simulink model "propeller"  (R2019b)
settings: Solver=VariableStepAuto  StartTime=0.0  StopTime=180  MaxStep=1e-2  RelTol=1e-3
undefined symbols (not defined in the file or in its folder): X, Y, Z
libraries: sm_lib x26, cstblocks x23, nesl_utility x20, simulink x2
(part 2 of 3)

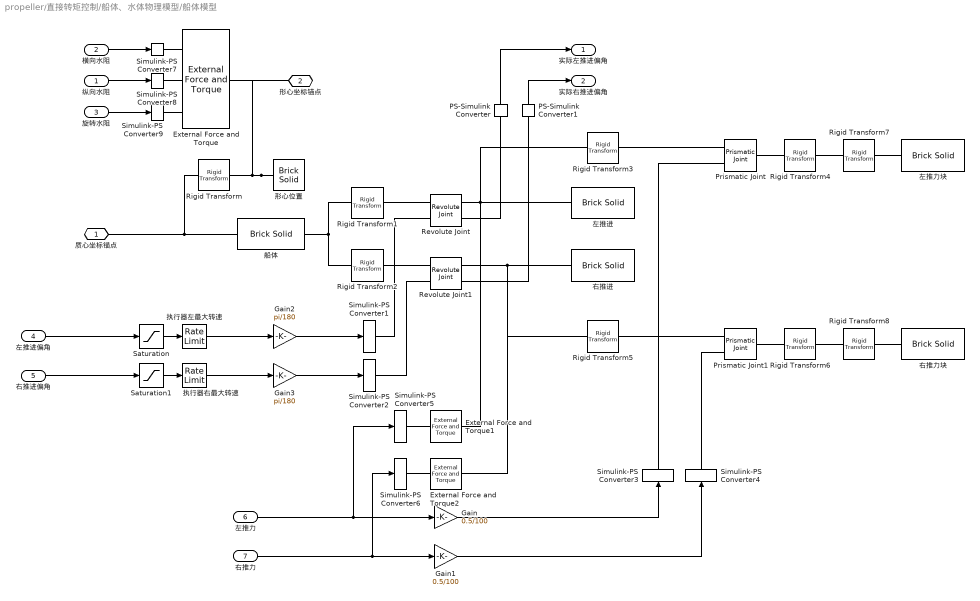
== system propeller/直接转矩控制/船体、水体物理模型/船体模型 ==
  纵向水阻 : Inport
  横向水阻 : Inport  Port=2
  旋转水阻 : Inport  Port=3
  左推进偏角 : Inport  Port=4
  右推进偏角 : Inport  Port=5
  左推力 : Inport  Port=6
  右推力 : Inport  Port=7
  External Force and Torque : sm_lib/Forces and Torques/External Force and Torque  ForceResolutionFrame=AttachedFrame  EnableForceX=on  EnableForceY=on  EnableForceZ=off  EnableForce=off  TorqueResolutionFrame=AttachedFrame  EnableTorqueX=off  EnableTorqueY=off  EnableTorqueZ=on  EnableTorque=off
  External Force and Torque1 : sm_lib/Forces and Torques/External Force and Torque  ForceResolutionFrame=AttachedFrame  EnableForceX=off  EnableForceY=on  EnableForceZ=off  EnableForce=off  TorqueResolutionFrame=AttachedFrame  EnableTorqueX=off  EnableTorqueY=off  EnableTorqueZ=off  EnableTorque=off
  External Force and Torque2 : sm_lib/Forces and Torques/External Force and Torque  ForceResolutionFrame=AttachedFrame  EnableForceX=off  EnableForceY=on  EnableForceZ=off  EnableForce=off  TorqueResolutionFrame=AttachedFrame  EnableTorqueX=off  EnableTorqueY=off  EnableTorqueZ=off  EnableTorque=off
  Gain : Gain  Gain=0.5/100
  Gain1 : Gain  Gain=0.5/100
  Gain2 : Gain  Gain=pi/180
  Gain3 : Gain  Gain=pi/180
  PS-Simulink Converter : nesl_utility/PS-Simulink Converter  PhysicalDomain=network_engine_domain  SubClassName=ps_output  LeftPortType=input  RightPortType=output  PseudoPeriodic=off  Frequencies=[]  Unit=inherit  AffineConversion=off
  PS-Simulink Converter1 : nesl_utility/PS-Simulink Converter  PhysicalDomain=network_engine_domain  SubClassName=ps_output  LeftPortType=input  RightPortType=output  PseudoPeriodic=off  Frequencies=[]  Unit=inherit  AffineConversion=off
  Prismatic Joint : sm_lib/Joints/Prismatic Joint  JointMode=Normal  SenseConstraintForce=off  SenseConstraintForceX=off  SenseConstraintForceY=off  SenseConstraintForceZ=off  SenseConstraintTorque=off  SenseConstraintTorqueX=off  SenseConstraintTorqueY=off  SenseConstraintTorqueZ=off  SenseTotalForce=off  SenseTotalForceX=off  SenseTotalForceY=off  SenseTotalForceZ=off  SenseTotalTorque=off  SenseTotalTorqueX=off  SenseTotalTorqueY=off  SenseTotalTorqueZ=off  CompositeWrenchDir=FollowerOnBase  CompositeWrenchFrame=BaseFrame  EquilibriumPosition=0  EquilibriumPositionUnits=m  SpringStiffness=0  SpringStiffnessUnits=N/m  DampingCoefficient=0  DampingCoefficientUnits=N/(m/s)  TorqueActuationMode=ComputedTorque  MotionActuationMode=InputMotion  SensePosition=off  SenseVelocity=off  SenseAcceleration=off  SenseTorqueForce=off  SenseLowerLimitTorqueForce=off  SenseUpperLimitTorqueForce=off  LowerLimitSpecify=off  LowerLimitBound=-1  LowerLimitBoundUnits=m  LowerLimitStiffness=1e6  LowerLimitStiffnessUnits=N/m  LowerLimitDamping=1e3  LowerLimitDampingUnits=N/(m/s)  LowerLimitTransitionRegionWidth=1e-4  LowerLimitTransitionRegionWidthUnits=m  UpperLimitSpecify=off  UpperLimitBound=1  UpperLimitBoundUnits=m  UpperLimitStiffness=1e6  UpperLimitStiffnessUnits=N/m  UpperLimitDamping=1e3  UpperLimitDampingUnits=N/(m/s)  UpperLimitTransitionRegionWidth=1e-4  UpperLimitTransitionRegionWidthUnits=m  PositionTargetSpecify=off  PositionTargetPriority=High  PositionTargetValue=0  PositionTargetValueUnits=m  VelocityTargetSpecify=off  VelocityTargetPriority=High  VelocityTargetValue=0  VelocityTargetValueUnits=m/s
  Prismatic Joint1 : sm_lib/Joints/Prismatic Joint  JointMode=Normal  SenseConstraintForce=off  SenseConstraintForceX=off  SenseConstraintForceY=off  SenseConstraintForceZ=off  SenseConstraintTorque=off  SenseConstraintTorqueX=off  SenseConstraintTorqueY=off  SenseConstraintTorqueZ=off  SenseTotalForce=off  SenseTotalForceX=off  SenseTotalForceY=off  SenseTotalForceZ=off  SenseTotalTorque=off  SenseTotalTorqueX=off  SenseTotalTorqueY=off  SenseTotalTorqueZ=off  CompositeWrenchDir=FollowerOnBase  CompositeWrenchFrame=BaseFrame  EquilibriumPosition=0  EquilibriumPositionUnits=m  SpringStiffness=0  SpringStiffnessUnits=N/m  DampingCoefficient=0  DampingCoefficientUnits=N/(m/s)  TorqueActuationMode=ComputedTorque  MotionActuationMode=InputMotion  SensePosition=off  SenseVelocity=off  SenseAcceleration=off  SenseTorqueForce=off  SenseLowerLimitTorqueForce=off  SenseUpperLimitTorqueForce=off  LowerLimitSpecify=off  LowerLimitBound=-1  LowerLimitBoundUnits=m  LowerLimitStiffness=1e6  LowerLimitStiffnessUnits=N/m  LowerLimitDamping=1e3  LowerLimitDampingUnits=N/(m/s)  LowerLimitTransitionRegionWidth=1e-4  LowerLimitTransitionRegionWidthUnits=m  UpperLimitSpecify=off  UpperLimitBound=1  UpperLimitBoundUnits=m  UpperLimitStiffness=1e6  UpperLimitStiffnessUnits=N/m  UpperLimitDamping=1e3  UpperLimitDampingUnits=N/(m/s)  UpperLimitTransitionRegionWidth=1e-4  UpperLimitTransitionRegionWidthUnits=m  PositionTargetSpecify=off  PositionTargetPriority=High  PositionTargetValue=0  PositionTargetValueUnits=m  VelocityTargetSpecify=off  VelocityTargetPriority=High  VelocityTargetValue=0  VelocityTargetValueUnits=m/s
  Revolute Joint : sm_lib/Joints/Revolute Joint  JointMode=Normal  SenseConstraintForce=off  SenseConstraintForceX=off  SenseConstraintForceY=off  SenseConstraintForceZ=off  SenseConstraintTorque=off  SenseConstraintTorqueX=off  SenseConstraintTorqueY=off  SenseConstraintTorqueZ=off  SenseTotalForce=off  SenseTotalForceX=off  SenseTotalForceY=off  SenseTotalForceZ=off  SenseTotalTorque=off  SenseTotalTorqueX=off  SenseTotalTorqueY=off  SenseTotalTorqueZ=off  CompositeWrenchDir=FollowerOnBase  CompositeWrenchFrame=BaseFrame  EquilibriumPosition=0  EquilibriumPositionUnits=deg  SpringStiffness=0  SpringStiffnessUnits=N*m/deg  DampingCoefficient=0  DampingCoefficientUnits=N*m/(deg/s)  TorqueActuationMode=ComputedTorque  MotionActuationMode=InputMotion  SensePosition=on  SenseVelocity=off  SenseAcceleration=off  SenseTorqueForce=off  SenseLowerLimitTorqueForce=off  SenseUpperLimitTorqueForce=off  LowerLimitSpecify=off  LowerLimitBound=-90  LowerLimitBoundUnits=deg  LowerLimitStiffness=1e4  LowerLimitStiffnessUnits=N*m/deg  LowerLimitDamping=10  LowerLimitDampingUnits=N*m/(deg/s)  LowerLimitTransitionRegionWidth=0.1  LowerLimitTransitionRegionWidthUnits=deg  UpperLimitSpecify=off  UpperLimitBound=90  UpperLimitBoundUnits=deg  UpperLimitStiffness=1e4  UpperLimitStiffnessUnits=N*m/deg  UpperLimitDamping=10  UpperLimitDampingUnits=N*m/(deg/s)  UpperLimitTransitionRegionWidth=0.1  UpperLimitTransitionRegionWidthUnits=deg  PositionTargetSpecify=off  PositionTargetPriority=High  PositionTargetValue=0  PositionTargetValueUnits=deg  VelocityTargetSpecify=off  VelocityTargetPriority=High  VelocityTargetValue=0  VelocityTargetValueUnits=deg/s
  Revolute Joint1 : sm_lib/Joints/Revolute Joint  JointMode=Normal  SenseConstraintForce=off  SenseConstraintForceX=off  SenseConstraintForceY=off  SenseConstraintForceZ=off  SenseConstraintTorque=off  SenseConstraintTorqueX=off  SenseConstraintTorqueY=off  SenseConstraintTorqueZ=off  SenseTotalForce=off  SenseTotalForceX=off  SenseTotalForceY=off  SenseTotalForceZ=off  SenseTotalTorque=off  SenseTotalTorqueX=off  SenseTotalTorqueY=off  SenseTotalTorqueZ=off  CompositeWrenchDir=FollowerOnBase  CompositeWrenchFrame=BaseFrame  EquilibriumPosition=0  EquilibriumPositionUnits=deg  SpringStiffness=0  SpringStiffnessUnits=N*m/deg  DampingCoefficient=0  DampingCoefficientUnits=N*m/(deg/s)  TorqueActuationMode=ComputedTorque  MotionActuationMode=InputMotion  SensePosition=on  SenseVelocity=off  SenseAcceleration=off  SenseTorqueForce=off  SenseLowerLimitTorqueForce=off  SenseUpperLimitTorqueForce=off  LowerLimitSpecify=off  LowerLimitBound=-90  LowerLimitBoundUnits=deg  LowerLimitStiffness=1e4  LowerLimitStiffnessUnits=N*m/deg  LowerLimitDamping=10  LowerLimitDampingUnits=N*m/(deg/s)  LowerLimitTransitionRegionWidth=0.1  LowerLimitTransitionRegionWidthUnits=deg  UpperLimitSpecify=off  UpperLimitBound=90  UpperLimitBoundUnits=deg  UpperLimitStiffness=1e4  UpperLimitStiffnessUnits=N*m/deg  UpperLimitDamping=10  UpperLimitDampingUnits=N*m/(deg/s)  UpperLimitTransitionRegionWidth=0.1  UpperLimitTransitionRegionWidthUnits=deg  PositionTargetSpecify=off  PositionTargetPriority=High  PositionTargetValue=0  PositionTargetValueUnits=deg  VelocityTargetSpecify=off  VelocityTargetPriority=High  VelocityTargetValue=0  VelocityTargetValueUnits=deg/s
  Rigid Transform : sm_lib/Frames and Transforms/Rigid Transform  TranslationMethod=Cartesian  TranslationStandardOffset=1  TranslationLengthUnit=m  TranslationStandardAxis=-Y  TranslationCartesianOffset=[0 -1 0]  TranslationROffset=0  TranslationROffsetUnits=m  TranslationZOffset=0  TranslationZOffsetUnits=m  TranslationThetaOffset=0  TranslationThetaOffsetUnits=deg  RotationMethod=None  RotationAngleUnits=deg  RotationStandardAxis=+Z  RotationAngle=0.0  RotationArbitraryAxis=[0 0 1]  FollAlignAxisA=+X  BaseAlignAxisA=+Y  FollAlignAxisB=+Y  BaseAlignAxisB=+Z  RotationSequenceAxes=FollowerAxes  RotationSequence=XYX  RotationSequenceAngles=[0 0 0]  RotationSequenceAnglesUnits=deg  RotationMatrix=[1 0 0; 0 1 0; 0 0 1]
  Rigid Transform1 : sm_lib/Frames and Transforms/Rigid Transform  TranslationMethod=Cartesian  TranslationStandardOffset=1  TranslationLengthUnit=m  TranslationStandardAxis=-Y  TranslationCartesianOffset=[-1 0 0]  TranslationROffset=0  TranslationROffsetUnits=m  TranslationZOffset=0  TranslationZOffsetUnits=m  TranslationThetaOffset=0  TranslationThetaOffsetUnits=deg  RotationMethod=None  RotationAngleUnits=deg  RotationStandardAxis=+Z  RotationAngle=0.0  RotationArbitraryAxis=[0 0 1]  FollAlignAxisA=+X  BaseAlignAxisA=+Y  FollAlignAxisB=+Y  BaseAlignAxisB=+Z  RotationSequenceAxes=FollowerAxes  RotationSequence=XYX  RotationSequenceAngles=[0 0 0]  RotationSequenceAnglesUnits=deg  RotationMatrix=[1 0 0; 0 1 0; 0 0 1]
  Rigid Transform2 : sm_lib/Frames and Transforms/Rigid Transform  TranslationMethod=Cartesian  TranslationStandardOffset=1  TranslationLengthUnit=m  TranslationStandardAxis=-Y  TranslationCartesianOffset=[1 0 0]  TranslationROffset=0  TranslationROffsetUnits=m  TranslationZOffset=0  TranslationZOffsetUnits=m  TranslationThetaOffset=0  TranslationThetaOffsetUnits=deg  RotationMethod=None  RotationAngleUnits=deg  RotationStandardAxis=+Z  RotationAngle=0.0  RotationArbitraryAxis=[0 0 1]  FollAlignAxisA=+X  BaseAlignAxisA=+Y  FollAlignAxisB=+Y  BaseAlignAxisB=+Z  RotationSequenceAxes=FollowerAxes  RotationSequence=XYX  RotationSequenceAngles=[0 0 0]  RotationSequenceAnglesUnits=deg  RotationMatrix=[1 0 0; 0 1 0; 0 0 1]
  Rigid Transform3 : sm_lib/Frames and Transforms/Rigid Transform  TranslationMethod=None  TranslationStandardOffset=1  TranslationLengthUnit=m  TranslationStandardAxis=-Y  TranslationCartesianOffset=[0 -1 0]  TranslationROffset=0  TranslationROffsetUnits=m  TranslationZOffset=0  TranslationZOffsetUnits=m  TranslationThetaOffset=0  TranslationThetaOffsetUnits=deg  RotationMethod=StandardAxis  RotationAngleUnits=deg  RotationStandardAxis=+X  RotationAngle=90  RotationArbitraryAxis=[0 0 1]  FollAlignAxisA=+X  BaseAlignAxisA=+Y  FollAlignAxisB=+Y  BaseAlignAxisB=+Z  RotationSequenceAxes=FollowerAxes  RotationSequence=XYX  RotationSequenceAngles=[0 0 0]  RotationSequenceAnglesUnits=deg  RotationMatrix=[1 0 0; 0 1 0; 0 0 1]
  Rigid Transform4 : sm_lib/Frames and Transforms/Rigid Transform  TranslationMethod=None  TranslationStandardOffset=1  TranslationLengthUnit=m  TranslationStandardAxis=-Y  TranslationCartesianOffset=[0 -1 0]  TranslationROffset=0  TranslationROffsetUnits=m  TranslationZOffset=0  TranslationZOffsetUnits=m  TranslationThetaOffset=0  TranslationThetaOffsetUnits=deg  RotationMethod=StandardAxis  RotationAngleUnits=deg  RotationStandardAxis=-X  RotationAngle=90  RotationArbitraryAxis=[0 0 1]  FollAlignAxisA=+X  BaseAlignAxisA=+Y  FollAlignAxisB=+Y  BaseAlignAxisB=+Z  RotationSequenceAxes=FollowerAxes  RotationSequence=XYX  RotationSequenceAngles=[0 0 0]  RotationSequenceAnglesUnits=deg  RotationMatrix=[1 0 0; 0 1 0; 0 0 1]
  Rigid Transform5 : sm_lib/Frames and Transforms/Rigid Transform  TranslationMethod=None  TranslationStandardOffset=1  TranslationLengthUnit=m  TranslationStandardAxis=-Y  TranslationCartesianOffset=[0 -1 0]  TranslationROffset=0  TranslationROffsetUnits=m  TranslationZOffset=0  TranslationZOffsetUnits=m  TranslationThetaOffset=0  TranslationThetaOffsetUnits=deg  RotationMethod=StandardAxis  RotationAngleUnits=deg  RotationStandardAxis=+X  RotationAngle=90  RotationArbitraryAxis=[0 0 1]  FollAlignAxisA=+X  BaseAlignAxisA=+Y  FollAlignAxisB=+Y  BaseAlignAxisB=+Z  RotationSequenceAxes=FollowerAxes  RotationSequence=XYX  RotationSequenceAngles=[0 0 0]  RotationSequenceAnglesUnits=deg  RotationMatrix=[1 0 0; 0 1 0; 0 0 1]
  Rigid Transform6 : sm_lib/Frames and Transforms/Rigid Transform  TranslationMethod=None  TranslationStandardOffset=1  TranslationLengthUnit=m  TranslationStandardAxis=-Y  TranslationCartesianOffset=[0 -1 0]  TranslationROffset=0  TranslationROffsetUnits=m  TranslationZOffset=0  TranslationZOffsetUnits=m  TranslationThetaOffset=0  TranslationThetaOffsetUnits=deg  RotationMethod=StandardAxis  RotationAngleUnits=deg  RotationStandardAxis=-X  RotationAngle=90  RotationArbitraryAxis=[0 0 1]  FollAlignAxisA=+X  BaseAlignAxisA=+Y  FollAlignAxisB=+Y  BaseAlignAxisB=+Z  RotationSequenceAxes=FollowerAxes  RotationSequence=XYX  RotationSequenceAngles=[0 0 0]  RotationSequenceAnglesUnits=deg  RotationMatrix=[1 0 0; 0 1 0; 0 0 1]
  Rigid Transform7 : sm_lib/Frames and Transforms/Rigid Transform  TranslationMethod=StandardAxis  TranslationStandardOffset=0.25  TranslationLengthUnit=m  TranslationStandardAxis=-Y  TranslationCartesianOffset=[0 -1 0]  TranslationROffset=0  TranslationROffsetUnits=m  TranslationZOffset=0  TranslationZOffsetUnits=m  TranslationThetaOffset=0  TranslationThetaOffsetUnits=deg  RotationMethod=None  RotationAngleUnits=deg  RotationStandardAxis=-X  RotationAngle=90  RotationArbitraryAxis=[0 0 1]  FollAlignAxisA=+X  BaseAlignAxisA=+Y  FollAlignAxisB=+Y  BaseAlignAxisB=+Z  RotationSequenceAxes=FollowerAxes  RotationSequence=XYX  RotationSequenceAngles=[0 0 0]  RotationSequenceAnglesUnits=deg  RotationMatrix=[1 0 0; 0 1 0; 0 0 1]
  Rigid Transform8 : sm_lib/Frames and Transforms/Rigid Transform  TranslationMethod=StandardAxis  TranslationStandardOffset=0.25  TranslationLengthUnit=m  TranslationStandardAxis=-Y  TranslationCartesianOffset=[0 -1 0]  TranslationROffset=0  TranslationROffsetUnits=m  TranslationZOffset=0  TranslationZOffsetUnits=m  TranslationThetaOffset=0  TranslationThetaOffsetUnits=deg  RotationMethod=None  RotationAngleUnits=deg  RotationStandardAxis=-X  RotationAngle=90  RotationArbitraryAxis=[0 0 1]  FollAlignAxisA=+X  BaseAlignAxisA=+Y  FollAlignAxisB=+Y  BaseAlignAxisB=+Z  RotationSequenceAxes=FollowerAxes  RotationSequence=XYX  RotationSequenceAngles=[0 0 0]  RotationSequenceAnglesUnits=deg  RotationMatrix=[1 0 0; 0 1 0; 0 0 1]
  Saturation : Saturate  UpperLimit=30  LowerLimit=-30
  Saturation1 : Saturate  UpperLimit=30  LowerLimit=-30
  Simulink-PS Converter{1..4} (4 alike) : nesl_utility/Simulink-PS Converter  PhysicalDomain=network_engine_domain  SubClassName=ps_input  LeftPortType=input  RightPortType=output  PseudoPeriodic=off  Frequencies=[]  NoiseDistribution=none  NoiseParameters=[]  Unit=1  AffineConversion=off  FilteringAndDerivatives=filter  SimscapeFilterOrder=2  InputFilterTimeConstant=0.01  UdotUserProvided=1
  Simulink-PS Converter{5..9} (5 alike) : nesl_utility/Simulink-PS Converter  PhysicalDomain=network_engine_domain  SubClassName=ps_input  LeftPortType=input  RightPortType=output  PseudoPeriodic=off  Frequencies=[]  NoiseDistribution=none  NoiseParameters=[]  Unit=1  AffineConversion=off  FilteringAndDerivatives=provide  SimscapeFilterOrder=2  InputFilterTimeConstant=0.01  UdotUserProvided=0
  右推力块 : sm_lib/Body Elements/Brick Solid  GraphicAmbientColor=[0.15 0.15 0.15 1.0]  BasedOnType=Mass  BrickDimensions=[0.15 0.05 0.15]  BrickDimensionUnits=m  CenterOfMass=[0 0 0]  CenterOfMassUnits=m  GraphicDiffuseColor=[0.8 0.0 0.0]  Density=1000  DensityUnits=kg/m^3  DoExposeReferenceFrame=off  GraphicEmissiveColor=[0.0 0.0 0.0 1.0]  ExportEntireGeometry=off  SerializedFrames=<Frames><Frame><Id>Frame1</Id><Value><Name>零位面</Name><Origin><Source>CenterOfMassFrame</Source><FeatureName></FeatureName></Origin><PrimaryAxis><DefinedDirection>+Z</DefinedDirection><Source>ReferenceFrame</Source><SourceDirection>+Z</SourceDirection><FeatureName></FeatureName></PrimaryAxis><SecondaryAxis><DefinedDirection>+X</DefinedDirection><Source>ReferenceFrame</Source><SourceDirection>+X</SourceDirection><FeatureName></FeatureName></SecondaryAxis></Value></Frame></Frames>  MarkerShape=Sphere  MarkerSize=10  GraphicType=FromGeometry  InertiaType=CalculateFromGeometry  Mass=0  MassUnits=kg  MomentsOfInertia=[1 1 1]  MomentsOfInertiaUnits=kg*m^2  GraphicOpacity=1  ProductsOfInertia=[0 0 0]  ProductsOfInertiaUnits=kg*m^2  GraphicShininess=75  GraphicSpecularColor=[0.5 0.5 0.5 1.0]  GraphicVisPropType=SimpleVisualProperties
  右推进 : sm_lib/Body Elements/Brick Solid  GraphicAmbientColor=[0.15 0.15 0.15 1.0]  BasedOnType=Mass  BrickDimensions=[0.2 0.5 0.2]  BrickDimensionUnits=m  CenterOfMass=[0 0 0]  CenterOfMassUnits=m  GraphicDiffuseColor=[0.6 0.6 1.0]  Density=1000  DensityUnits=kg/m^3  DoExposeReferenceFrame=off  GraphicEmissiveColor=[0.0 0.0 0.0 1.0]  ExportEntireGeometry=off  SerializedFrames=<Frames><Frame><Id>Frame1</Id><Value><Name>转轴</Name><Origin><Source>GeometricFeature</Source><FeatureName>+y surface</FeatureName></Origin><PrimaryAxis><DefinedDirection>+Z</DefinedDirection><Source>ReferenceFrame</Source><SourceDirection>+Z</SourceDirection><FeatureName></FeatureName></PrimaryAxis><SecondaryAxis><DefinedDirection>+X</DefinedDirection><Source>ReferenceFrame</Source><SourceDirection>+X</SourceDirection><FeatureName></FeatureName></SecondaryAxis></Value></Frame></Frames>  MarkerShape=Sphere  MarkerSize=10  GraphicType=FromGeometry  InertiaType=CalculateFromGeometry  Mass=0  MassUnits=kg  MomentsOfInertia=[1 1 1]  MomentsOfInertiaUnits=kg*m^2  GraphicOpacity=0.3  ProductsOfInertia=[0 0 0]  ProductsOfInertiaUnits=kg*m^2  GraphicShininess=75  GraphicSpecularColor=[0.5 0.5 0.5 1.0]  GraphicVisPropType=SimpleVisualProperties
  左推力块 : sm_lib/Body Elements/Brick Solid  GraphicAmbientColor=[0.15 0.15 0.15 1.0]  BasedOnType=Mass  BrickDimensions=[0.15 0.05 0.15]  BrickDimensionUnits=m  CenterOfMass=[0 0 0]  CenterOfMassUnits=m  GraphicDiffuseColor=[0.8 0.0 0.0]  Density=1000  DensityUnits=kg/m^3  DoExposeReferenceFrame=off  GraphicEmissiveColor=[0.0 0.0 0.0 1.0]  ExportEntireGeometry=off  SerializedFrames=<Frames><Frame><Id>Frame1</Id><Value><Name>零位面</Name><Origin><Source>CenterOfMassFrame</Source><FeatureName></FeatureName></Origin><PrimaryAxis><DefinedDirection>+Z</DefinedDirection><Source>ReferenceFrame</Source><SourceDirection>+Z</SourceDirection><FeatureName></FeatureName></PrimaryAxis><SecondaryAxis><DefinedDirection>+X</DefinedDirection><Source>ReferenceFrame</Source><SourceDirection>+X</SourceDirection><FeatureName></FeatureName></SecondaryAxis></Value></Frame></Frames>  MarkerShape=Sphere  MarkerSize=10  GraphicType=FromGeometry  InertiaType=CalculateFromGeometry  Mass=0  MassUnits=kg  MomentsOfInertia=[1 1 1]  MomentsOfInertiaUnits=kg*m^2  GraphicOpacity=1  ProductsOfInertia=[0 0 0]  ProductsOfInertiaUnits=kg*m^2  GraphicShininess=75  GraphicSpecularColor=[0.5 0.5 0.5 1.0]  GraphicVisPropType=SimpleVisualProperties
  左推进 : sm_lib/Body Elements/Brick Solid  GraphicAmbientColor=[0.15 0.15 0.15 1.0]  BasedOnType=Mass  BrickDimensions=[0.2 0.5 0.2]  BrickDimensionUnits=m  CenterOfMass=[0 0 0]  CenterOfMassUnits=m  GraphicDiffuseColor=[0.6 0.6 1.0]  Density=1000  DensityUnits=kg/m^3  DoExposeReferenceFrame=off  GraphicEmissiveColor=[0.0 0.0 0.0 1.0]  ExportEntireGeometry=off  SerializedFrames=<Frames><Frame><Id>Frame1</Id><Value><Name>转轴</Name><Origin><Source>GeometricFeature</Source><FeatureName>+y surface</FeatureName></Origin><PrimaryAxis><DefinedDirection>+Z</DefinedDirection><Source>ReferenceFrame</Source><SourceDirection>+Z</SourceDirection><FeatureName></FeatureName></PrimaryAxis><SecondaryAxis><DefinedDirection>+X</DefinedDirection><Source>ReferenceFrame</Source><SourceDirection>+X</SourceDirection><FeatureName></FeatureName></SecondaryAxis></Value></Frame></Frames>  MarkerShape=Sphere  MarkerSize=10  GraphicType=FromGeometry  InertiaType=CalculateFromGeometry  Mass=0  MassUnits=kg  MomentsOfInertia=[1 1 1]  MomentsOfInertiaUnits=kg*m^2  GraphicOpacity=0.3  ProductsOfInertia=[0 0 0]  ProductsOfInertiaUnits=kg*m^2  GraphicShininess=75  GraphicSpecularColor=[0.5 0.5 0.5 1.0]  GraphicVisPropType=SimpleVisualProperties
  形心位置 : sm_lib/Body Elements/Brick Solid  GraphicAmbientColor=[0.15 0.15 0.15 1.0]  BasedOnType=Mass  BrickDimensions=[0.2 0.2 0.2]  BrickDimensionUnits=m  CenterOfMass=[0 0 0]  CenterOfMassUnits=m  GraphicDiffuseColor=[0.0 0.0 0.8]  Density=1000  DensityUnits=kg/m^3  DoExposeReferenceFrame=on  GraphicEmissiveColor=[0.0 0.0 0.0 1.0]  ExportEntireGeometry=off  SerializedFrames=<Frames/>  MarkerShape=Sphere  MarkerSize=10  GraphicType=FromGeometry  InertiaType=CalculateFromGeometry  Mass=0  MassUnits=kg  MomentsOfInertia=[1 1 1]  MomentsOfInertiaUnits=kg*m^2  GraphicOpacity=0.8  ProductsOfInertia=[0 0 0]  ProductsOfInertiaUnits=kg*m^2  GraphicShininess=75  GraphicSpecularColor=[0.5 0.5 0.5 1.0]  GraphicVisPropType=SimpleVisualProperties
  执行器右最大转速 : RateLimiter  RisingSlewLimit=15  FallingSlewLimit=-15  SampleTimeMode=inherited
  执行器左最大转速 : RateLimiter  RisingSlewLimit=15  FallingSlewLimit=-15  SampleTimeMode=inherited
  船体 : sm_lib/Body Elements/Brick Solid  GraphicAmbientColor=[0.15 0.15 0.15 1.0]  BasedOnType=Mass  BrickDimensions=[3 6 0.5]  BrickDimensionUnits=m  CenterOfMass=[0 0 0]  CenterOfMassUnits=m  GraphicDiffuseColor=[0.0 0.8 0.8]  Density=1000  DensityUnits=kg/m^3  DoExposeReferenceFrame=on  GraphicEmissiveColor=[0.0 0.0 0.0 1.0]  ExportEntireGeometry=off  SerializedFrames=<Frames><Frame><Id>Frame1</Id><Value><Name>船尾</Name><Origin><Source>GeometricFeature</Source><FeatureName>-y surface</FeatureName></Origin><PrimaryAxis><DefinedDirection>+Z</DefinedDirection><Source>ReferenceFrame</Source><SourceDirection>+Z</SourceDirection><FeatureName></FeatureName></PrimaryAxis><SecondaryAxis><DefinedDirection>+X</DefinedDirection><Source>ReferenceFrame</Source><SourceDirection>+X</SourceDirection><FeatureName></FeatureName></SecondaryAxis></Value></Frame></Frames>  MarkerShape=Sphere  MarkerSize=10  GraphicType=FromGeometry  InertiaType=CalculateFromGeometry  Mass=M_Set  MassUnits=kg  MomentsOfInertia=[1 1 1]  MomentsOfInertiaUnits=kg*m^2  GraphicOpacity=0.7  ProductsOfInertia=[0 0 0]  ProductsOfInertiaUnits=kg*m^2  GraphicShininess=75  GraphicSpecularColor=[0.5 0.5 0.5 1.0]  GraphicVisPropType=SimpleVisualProperties
  质心坐标锚点 : PMIOPort  Side=Left
  形心坐标锚点 : PMIOPort  Port=2  Side=Left
  实际左推进偏角 : Outport
  实际右推进偏角 : Outport  Port=2
  wires:
  右推力/1 -> Simulink-PS Converter6/1, Gain1/1
  Gain/1 -> Simulink-PS Converter3/1
  Gain3/1 -> Simulink-PS Converter2/1
  Gain2/1 -> Simulink-PS Converter1/1
  Gain1/1 -> Simulink-PS Converter4/1
  左推力/1 -> Simulink-PS Converter5/1, Gain/1
  旋转水阻/1 -> Simulink-PS Converter9/1
  纵向水阻/1 -> Simulink-PS Converter8/1
  横向水阻/1 -> Simulink-PS Converter7/1
  PS-Simulink Converter1/1 -> 实际右推进偏角/1
  PS-Simulink Converter/1 -> 实际左推进偏角/1
  左推进偏角/1 -> Saturation/1
  Saturation1/1 -> 执行器右最大转速/1
  Saturation/1 -> 执行器左最大转速/1
  执行器左最大转速/1 -> Gain2/1
  右推进偏角/1 -> Saturation1/1
  执行器右最大转速/1 -> Gain3/1
  connections:
  Revolute Joint/LConn1 -- Rigid Transform1/RConn1
  Simulink-PS Converter5/RConn1 -- External Force and Torque1/LConn1
  Revolute Joint/RConn1 -- External Force and Torque1/RConn1 -- Rigid Transform3/LConn1 -- 左推进/LConn1
  Rigid Transform1/LConn1 -- Rigid Transform2/LConn1 -- 船体/LConn1
  Revolute Joint1/RConn1 -- Rigid Transform5/LConn1 -- External Force and Torque2/RConn1 -- 右推进/LConn1
  形心位置/RConn1 -- 形心坐标锚点/RConn1 -- External Force and Torque/RConn1 -- Rigid Transform/RConn1
  Rigid Transform7/RConn1 -- 左推力块/LConn1
  Prismatic Joint/LConn1 -- Rigid Transform3/RConn1
  Simulink-PS Converter2/RConn1 -- Revolute Joint1/LConn2
  Revolute Joint1/LConn1 -- Rigid Transform2/RConn1
  Simulink-PS Converter7/RConn1 -- External Force and Torque/LConn1
  Simulink-PS Converter8/RConn1 -- External Force and Torque/LConn2
  External Force and Torque2/LConn1 -- Simulink-PS Converter6/RConn1
  右推力块/LConn1 -- Rigid Transform8/RConn1
  船体/RConn1 -- 质心坐标锚点/RConn1 -- Rigid Transform/LConn1
  Rigid Transform4/LConn1 -- Prismatic Joint/RConn1
  Prismatic Joint1/LConn1 -- Rigid Transform5/RConn1
  Simulink-PS Converter9/RConn1 -- External Force and Torque/LConn3
  Rigid Transform6/LConn1 -- Prismatic Joint1/RConn1
  Simulink-PS Converter1/RConn1 -- Revolute Joint/LConn2
  Simulink-PS Converter3/RConn1 -- Prismatic Joint/LConn2
  Prismatic Joint1/LConn2 -- Simulink-PS Converter4/RConn1
  Rigid Transform8/LConn1 -- Rigid Transform6/RConn1
  Rigid Transform7/LConn1 -- Rigid Transform4/RConn1
  PS-Simulink Converter/LConn1 -- Revolute Joint/RConn2
  PS-Simulink Converter1/LConn1 -- Revolute Joint1/RConn2

== system propeller/直接转矩控制/船速、朝向控制器/前进速度控制 ==
  速度反馈 : Inport
  速度设定 : Inport  Port=2
  Kd : Gain  Gain=Kd
  Ki : Gain  Gain=Ki
  Kp : Gain  Gain=Kp
  Product : Product  Inputs=**
  Saturation : Saturate  UpperLimit=Trq_p  LowerLimit=-Trq_n
  Sum : Sum  Inputs=|+-
  Sum1 : Sum  Inputs=+++
  Zero-Order Hold : ZeroOrderHold  SampleTime=0.01
  微分 : Subsystem  mask{fc_Set=D_Fc}
      mask prompts: fc_Set "截止频率（fc）"
  积分:限制正扭矩 : Integrator  LimitOutput=on  UpperSaturationLimit=Trq_p  LowerSaturationLimit=-Trq_n
  积分控制 : Subsystem  mask{dSpe=0.5}
      mask prompts: dSpe "停止积分的速度斜率 m/s2"
  前进力输出 : Outport
  wires:
  Kd/1 -> 微分/1(Err)
  微分/1(dErr) -> Sum1/3
  积分控制/1(开启积分) -> Product/2
  Sum/1 -> 积分控制/1(Error), Kd/1, Ki/1, Kp/1  "Error"
  Ki/1 -> Product/1
  Product/1 -> 积分:限制正扭矩/1
  Saturation/1 -> 前进力输出/1
  积分:限制正扭矩/1 -> Sum1/2
  Kp/1 -> Sum1/1
  速度设定/1 -> Sum/1
  速度反馈/1 -> Sum/2
  Sum1/1 -> 积分控制/2(Output), Zero-Order Hold/1
  Zero-Order Hold/1 -> Saturation/1

== system propeller/直接转矩控制/船速、朝向控制器/右电机控制 ==
  转速反馈 : Inport
  推力设定 : Inport  Port=2
  Sum1 : Sum  Inputs=|++
  补偿系数 : Gain  Gain=0.5
  角加速度补偿 : Subsystem  mask{Max_Acc=1000}
      mask prompts: Max_Acc "最大角加速度补偿量 Rpm/s"
  设定扭矩 : Outport
  wires:
  Sum1/1 -> 设定扭矩/1
  转速反馈/1 -> 角加速度补偿/1(转速反馈)
  补偿系数/1 -> Sum1/2
  角加速度补偿/1(加速消耗的扭矩) -> 补偿系数/1
  推力设定/1 -> Sum1/1

== system propeller/直接转矩控制/船速、朝向控制器/左电机控制 ==
  转速反馈 : Inport
  推力设定 : Inport  Port=2
  Sum1 : Sum  Inputs=|++
  补偿系数 : Gain  Gain=0.5
  角加速度补偿 : Subsystem  mask{Max_Acc=1000}
      mask prompts: Max_Acc "最大角加速度补偿量 Rpm/s"
  设定扭矩 : Outport
  wires:
  推力设定/1 -> Sum1/1
  角加速度补偿/1(加速消耗的扭矩) -> 补偿系数/1
  补偿系数/1 -> Sum1/2
  转速反馈/1 -> 角加速度补偿/1(转速反馈)
  Sum1/1 -> 设定扭矩/1

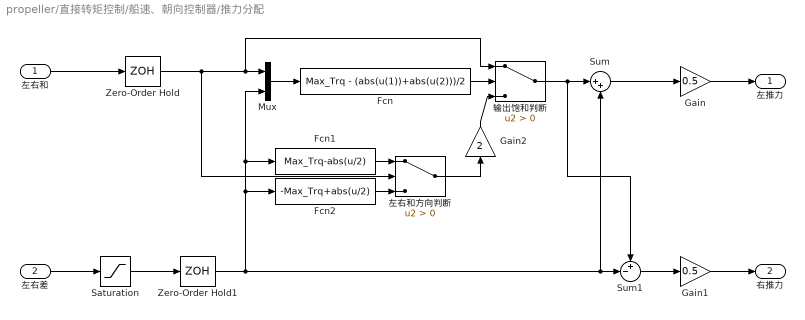
== system propeller/直接转矩控制/船速、朝向控制器/推力分配 ==
  左右和 : Inport
  左右差 : Inport  Port=2
  Fcn : Fcn  Expr=Max_Trq - (abs(u(1))+abs(u(2)))/2
  Fcn1 : Fcn  Expr=Max_Trq-abs(u/2)
  Fcn2 : Fcn  Expr=-Max_Trq+abs(u/2)
  Gain : Gain  Gain=0.5
  Gain1 : Gain  Gain=0.5
  Gain2 : Gain  Gain=2
  Mux : Mux  Inputs=2
  Saturation : Saturate  UpperLimit=Max_Trq*2  LowerLimit=-Max_Trq*2
  Sum : Sum  Inputs=|++
  Sum1 : Sum  Inputs=+-|
  Zero-Order Hold : ZeroOrderHold  SampleTime=0.01
  Zero-Order Hold1 : ZeroOrderHold  SampleTime=0.01
  左右和方向判断 : Switch  Criteria=u2 > Threshold
  输出饱和判断 : Switch  Criteria=u2 > Threshold
  左推力 : Outport
  右推力 : Outport  Port=2
  wires:
  左右差/1 -> Saturation/1
  Sum/1 -> Gain/1
  Gain/1 -> 左推力/1
  Gain1/1 -> 右推力/1
  Sum1/1 -> Gain1/1
  Fcn/1 -> 输出饱和判断/2
  左右和/1 -> Zero-Order Hold/1
  Mux/1 -> Fcn/1
  Saturation/1 -> Zero-Order Hold1/1
  输出饱和判断/1 -> Sum1/1, Sum/1
  左右和方向判断/1 -> Gain2/1
  Gain2/1 -> 输出饱和判断/3
  Fcn1/1 -> 左右和方向判断/1
  Fcn2/1 -> 左右和方向判断/3
  Zero-Order Hold/1 -> 左右和方向判断/2, 输出饱和判断/1, Mux/1
  Zero-Order Hold1/1 -> Fcn2/1, Mux/2, Fcn1/1, Sum/2, Sum1/2

== system propeller/直接转矩控制/船速、朝向控制器/推力解算 ==
  前进力 : Inport
  转向扭矩 : Inport  Port=2
  左右推进偏角 : Inport  Port=3
  Demux : Demux  Outputs=2
  Demux1 : Demux  Outputs=2
  If1 : If  IfExpression=u1 < 1e-6
  Memory : Memory
  Merge : Merge
  Mux : Mux  Inputs=6
  Th0 : Constant  Value=atan(a/b)
  Zero-Order Hold : ZeroOrderHold  SampleTime=0.01
  Zero-Order Hold1 : ZeroOrderHold  SampleTime=0.01
  c : Constant  Value=sqrt(a^2+b^2)
  扭矩无解 : Subsystem  TreatAsAtomicUnit=on
  扭矩无解检查 : Fcn  Expr=abs(u(5)+u(3)) + abs(u(5)-u(4))
  扭矩有解 : Subsystem
  左推力 : Outport
  右推力 : Outport  Port=2
  wires:
  Mux/1 -> Zero-Order Hold/1
  前进力/1 -> Mux/1
  转向扭矩/1 -> Mux/2
  Demux/1 -> 左推力/1
  Demux/2 -> 右推力/1
  Demux1/2 -> Mux/4
  Demux1/1 -> Mux/3
  左右推进偏角/1 -> Demux1/1
  c/1 -> Mux/6
  Th0/1 -> Mux/5
  Memory/1 -> Demux/1
  扭矩无解检查/1 -> If1/1
  Zero-Order Hold/1 -> 扭矩有解/1(状态输入), 扭矩无解/1(In1), 扭矩无解检查/1  "状态输入"
  If1/1 -> 扭矩无解/Action
  If1/2 -> 扭矩有解/Action
  Merge/1 -> Zero-Order Hold1/1
  扭矩无解/1(Out1) -> Merge/1
  扭矩有解/1(推力输出) -> Merge/2
  Zero-Order Hold1/1 -> Memory/1

== system propeller/直接转矩控制/船速、朝向控制器/方向分配 ==
  左右和 : Inport
  左右差 : Inport  Port=2
  Fcn : Fcn  Expr=Max_Th - (abs(u(1))+abs(u(2)))/2
  Fcn1 : Fcn  Expr=Max_Th-abs(u/2)
  Fcn2 : Fcn  Expr=-Max_Th+abs(u/2)
  Gain : Gain  Gain=0.5
  Gain1 : Gain  Gain=0.5
  Gain2 : Gain  Gain=2
  Mux : Mux  Inputs=2
  Saturation : Saturate  UpperLimit=Max_Th*2  LowerLimit=-Max_Th*2
  Sum : Sum  Inputs=|++
  Sum1 : Sum  Inputs=+-|
  左右和方向判断 : Switch  Criteria=u2 > Threshold
  输出饱和判断 : Switch  Criteria=u2 > Threshold
  左方向 : Outport
  右方向 : Outport  Port=2
  wires:
  左右差/1 -> Saturation/1
  Sum/1 -> Gain/1
  Gain/1 -> 左方向/1
  Gain1/1 -> 右方向/1
  Sum1/1 -> Gain1/1
  Fcn/1 -> 输出饱和判断/2
  左右和/1 -> 左右和方向判断/2, 输出饱和判断/1, Mux/1
  Mux/1 -> Fcn/1
  Saturation/1 -> Fcn2/1, Mux/2, Fcn1/1, Sum/2, Sum1/2
  输出饱和判断/1 -> Sum1/1, Sum/1
  左右和方向判断/1 -> Gain2/1
  Gain2/1 -> 输出饱和判断/3
  Fcn1/1 -> 左右和方向判断/1
  Fcn2/1 -> 左右和方向判断/3

== system propeller/直接转矩控制/船速、朝向控制器/舵内缩指令 ==
  设定前进力 : Inport
  设定扭矩 : Inport  Port=2
  Abs : Abs
  Constant : Constant  Value=Fy_Start
  Gain2 : Gain  Gain=180/pi
  If : If  IfExpression=u1 < 0
  If Action Subsystem : Subsystem  TreatAsAtomicUnit=on
  Memory : Memory
  Memory1 : Memory
  Memory2 : Memory
  Merge : Merge
  Subsystem : Subsystem
  Sum : Sum  Inputs=|+-
  Zero-Order Hold : ZeroOrderHold  SampleTime=0.05
  Zero-Order Hold1 : ZeroOrderHold  SampleTime=0.05
  Zero-Order Hold2 : ZeroOrderHold  SampleTime=0.05
  左右角度差 : Outport
  wires:
  Constant/1 -> Sum/2
  Sum/1 -> If/1
  Merge/1 -> Gain2/1
  If Action Subsystem/1(Out1) -> Merge/1
  Subsystem/1(左右差) -> Merge/2
  If/2 -> If Action Subsystem/Action
  If/1 -> Subsystem/Action
  Abs/1 -> Sum/1
  Memory1/1 -> Subsystem/2(转向扭矩)
  Memory/1 -> Subsystem/1(前进力), Abs/1
  Zero-Order Hold1/1 -> Memory1/1
  Zero-Order Hold/1 -> Memory/1
  设定扭矩/1 -> Zero-Order Hold1/1
  设定前进力/1 -> Zero-Order Hold/1
  Zero-Order Hold2/1 -> Memory2/1
  Memory2/1 -> 左右角度差/1
  Gain2/1 -> Zero-Order Hold2/1

== system propeller/直接转矩控制/船速、朝向控制器/舵朝向指令 ==
  设定前进力 : Inport
  设定扭矩 : Inport  Port=2
  Abs : Abs
  Constant : Constant  Value=Fy_Start
  Gain2 : Gain  Gain=180/pi
  If : If
  If Action Subsystem : Subsystem  TreatAsAtomicUnit=on
  Memory : Memory
  Memory1 : Memory
  Merge : Merge
  Subsystem : Subsystem
  Sum : Sum  Inputs=|+-
  Zero-Order Hold : ZeroOrderHold  SampleTime=0.05
  Zero-Order Hold1 : ZeroOrderHold  SampleTime=0.05
  左右角度和 : Outport
  wires:
  设定前进力/1 -> Zero-Order Hold/1
  设定扭矩/1 -> Zero-Order Hold1/1
  Zero-Order Hold/1 -> Memory/1
  Zero-Order Hold1/1 -> Memory1/1
  Gain2/1 -> 左右角度和/1
  Memory/1 -> Abs/1, Subsystem/1(前进力)
  Memory1/1 -> Subsystem/2(转向扭矩)
  Abs/1 -> Sum/1
  If/1 -> Subsystem/Action
  If/2 -> If Action Subsystem/Action
  Subsystem/1(左右和) -> Merge/2
  If Action Subsystem/1(Out1) -> Merge/1
  Merge/1 -> Gain2/1
  Sum/1 -> If/1
  Constant/1 -> Sum/2

== system propeller/直接转矩控制/船速、朝向控制器/船头方向PID ==
  角度反馈 : Inport
  角度设定 : Inport  Port=2
  Gain : Gain  Gain=pi/180
  Kd : Gain  Gain=Kd
  Ki : Gain  Gain=Ki
  Kp : Gain  Gain=Kp
  Product : Product  Inputs=**
  Saturation : Saturate  UpperLimit=Spe_p  LowerLimit=-Spe_n
  Scope : Scope
  Sum : Sum  Inputs=|+-
  Sum1 : Sum  Inputs=+++
  Transport Delay : TransportDelay  DelayTime=0.01
  反馈量滤波 : Subsystem  mask{Frq=D_Fc*3, Order=3}
      mask prompts: Frq "Frq_Set"; Order "Order_Set"
  微分 : Subsystem  mask{fc_Set=D_Fc}
      mask prompts: fc_Set "截止频率（fc）"
  积分:限制正扭矩 : Integrator  LimitOutput=on  UpperSaturationLimit=Spe_p  LowerSaturationLimit=-Spe_n
  积分控制 : Subsystem  mask{dAng=10}
      mask prompts: dAng "停止积分的角速度斜率 dps"
  角速度 : Outport
  wires:
  Saturation/1 -> Transport Delay/1
  Sum1/1 -> Saturation/1, 积分控制/2(Output)
  角度反馈/1 -> Sum/2
  角度设定/1 -> Sum/1
  Kp/1 -> Sum1/1
  积分:限制正扭矩/1 -> Sum1/2
  Transport Delay/1 -> 反馈量滤波/1(Signal)
  Product/1 -> 积分:限制正扭矩/1
  Ki/1 -> Product/1
  Sum/1 -> Kp/1, Ki/1, Kd/1, 积分控制/1(Error)  "Error"
  积分控制/1(开启积分) -> Product/2
  微分/1(dErr) -> Sum1/3, Scope/1
  Kd/1 -> 微分/1(Err)
  Gain/1 -> 角速度/1
  反馈量滤波/1(Output) -> Gain/1

== system propeller/直接转矩控制/船速、朝向控制器/设定值滤波 ==
  Signal : Inport
  Constant2 : Constant  Value=Frq
  Gain : Gain  Gain=2*pi
  d_Smp_LPF6 : cstblocks/Linear Parameter Varying/Varying Lowpass Filter  N=Order
      settings: SourceProductName=Control System Toolbox
  Output : Outport
  wires:
  Gain/1 -> d_Smp_LPF6/2
  Signal/1 -> d_Smp_LPF6/1
  Constant2/1 -> Gain/1
  d_Smp_LPF6/1 -> Output/1  "Is"

== system propeller/失败的水流估计模型/水流状态估计/螺旋桨状态模拟/If Action Subsystem ==
  In1 : Inport
  Action Port : ActionPort  ActionPortLabel=else
  Fcn2 : Fcn  Expr=u(1)/(sqrt(u(2)))
  Out1 : Outport
  wires:
  Fcn2/1 -> Out1/1
  In1/1 -> Fcn2/1

== system propeller/失败的水流估计模型/水流状态估计/螺旋桨状态模拟/If Action Subsystem1 ==
  In1 : Inport
  Action Port : ActionPort  ActionPortLabel=if(u1 < 1e-6)
  Fcn2 : Fcn  Expr=abs(u(1))
  Out1 : Outport
  wires:
  In1/1 -> Fcn2/1
  Fcn2/1 -> Out1/1

== system propeller/失败的水流估计模型/水流状态估计/螺旋桨状态模拟/螺旋桨工作特性表 ==
  J' : Inport
  转速 : Inport  Port=2
  If Action Subsystem2 : Subsystem  TreatAsAtomicUnit=on
  If Action Subsystem3 : Subsystem  TreatAsAtomicUnit=on
  If1 : If
  Merge1 : Merge
  Merge2 : Merge
  Kt : Outport
  Kq : Outport  Port=2
  wires:
  If Action Subsystem2/2(Kq) -> Merge2/1
  Merge2/1 -> Kq/1
  If Action Subsystem3/2(Kq) -> Merge2/2
  If Action Subsystem3/1(Kt) -> Merge1/2
  Merge1/1 -> Kt/1
  J'/1 -> If Action Subsystem2/1(J'), If Action Subsystem3/1(J')
  If Action Subsystem2/1(Kt) -> Merge1/1
  转速/1 -> If1/1
  If1/2 -> If Action Subsystem3/Action
  If1/1 -> If Action Subsystem2/Action

== system propeller/失败的水流估计模型/水流状态估计/螺旋桨状态模拟/螺旋桨工作特性表Backup ==
  J' : Inport
  转速 : Inport  Port=2
  If Action Subsystem2 : Subsystem  TreatAsAtomicUnit=on
  If Action Subsystem3 : Subsystem  TreatAsAtomicUnit=on
  If1 : If
  Merge1 : Merge
  Merge2 : Merge
  Kt : Outport
  Kq : Outport  Port=2
  wires:
  If1/1 -> If Action Subsystem2/Action
  If1/2 -> If Action Subsystem3/Action
  转速/1 -> If1/1
  If Action Subsystem2/1(Kt) -> Merge1/1
  J'/1 -> If Action Subsystem3/1(J'), If Action Subsystem2/1(J')
  Merge1/1 -> Kt/1
  If Action Subsystem3/1(Kt) -> Merge1/2
  If Action Subsystem3/2(Kq) -> Merge2/2
  Merge2/1 -> Kq/1
  If Action Subsystem2/2(Kq) -> Merge2/1

== system propeller/失败的水流估计模型/螺旋桨模型/螺旋桨工作特性表/If Action Subsystem2 ==
  J' : Inport
  Action Port : ActionPort  ActionPortLabel=if(u1 > 0)
  n+::Kq-扭矩系数 : Lookup_n-D  NumberOfTableDimensions=1  BreakpointsForDimension1=[-1,-0.9,-0.8,-0.7,-0.6,-0.5,-0.4,-0.3,-0.2,-0.1,0,0.1,0.2,0.3,0.4,0.5,0.6,0.7,0.8,0.9,1]  BreakpointsForDimension2=[1:3]  Table=[0.019242,0.038636,0.046717,0.049444,0.048333,0.043384,0.043081,0.045202,0.049242,0.051465,0.05197,0.050556,0.046111,0.040556,0.033081,0.024596,0.015543,0.0059848,-0.0059091,-0.013687,-0.016818]  InternalRulePriority=Speed  RndMeth=Simplest  InputSameDT=on
  n+::Kt-推力系数 : Lookup_n-D  NumberOfTableDimensions=1  BreakpointsForDimension1=[-1,-0.9,-0.8,-0.7,-0.6,-0.5,-0.4,-0.3,-0.2,-0.1,0,0.1,0.2,0.3,0.4,0.5,0.6,0.7,0.8,0.9,1]  BreakpointsForDimension2=[1:3]  Table=[0.082134,0.19766,0.30499,0.32898,0.31256,0.2589,0.25511,0.28226,0.35107,0.3738,0.38,0.36686,0.32645,0.26016,0.18188,0.10423,0.04173,-0.018245,-0.05423,-0.065593,-0.06]  InternalRulePriority=Speed  RndMeth=Simplest  InputSameDT=on
  Kt : Outport
  Kq : Outport  Port=2
  wires:
  n+::Kq-扭矩系数/1 -> Kq/1
  n+::Kt-推力系数/1 -> Kt/1
  J'/1 -> n+::Kq-扭矩系数/1, n+::Kt-推力系数/1

== system propeller/失败的水流估计模型/螺旋桨模型/螺旋桨工作特性表/If Action Subsystem3 ==
  J' : Inport
  Action Port : ActionPort  ActionPortLabel=else
  n-::Kq-扭矩系数 : Lookup_n-D  NumberOfTableDimensions=1  BreakpointsForDimension1=[-1,-0.9,-0.8,-0.7,-0.6,-0.5,-0.4,-0.3,-0.2,-0.1,0,0.1,0.2,0.3,0.4,0.5,0.6,0.7,0.8,0.9,1]  BreakpointsForDimension2=[1:3]  Table=[0.019242,0.016111,0.010354,-0.00035354,-0.014293,-0.025707,-0.034495,-0.041263,-0.046515,-0.051162,-0.05197,-0.051465,-0.049242,-0.045202,-0.043081,-0.043384,-0.04702,-0.049343,-0.045909,-0.038434,-0.016818]  InternalRulePriority=Speed  RndMeth=Simplest  InputSameDT=on
  n-::Kt-推力系数 : Lookup_n-D  NumberOfTableDimensions=1  BreakpointsForDimension1=[-1,-0.9,-0.8,-0.7,-0.6,-0.5,-0.4,-0.3,-0.2,-0.1,0,0.1,0.2,0.3,0.4,0.5,0.6,0.7,0.8,0.9,1]  BreakpointsForDimension2=[1:3]  Table=[0.082134,0.088952,0.080745,0.052336,-0.020896,-0.090341,-0.16989,-0.25764,-0.32014,-0.34981,-0.35676,-0.35549,-0.33409,-0.29015,-0.25379,-0.24924,-0.30379,-0.32197,-0.2947,-0.21894,-0.06]  InternalRulePriority=Speed  RndMeth=Simplest  InputSameDT=on
  Kt : Outport
  Kq : Outport  Port=2
  wires:
  J'/1 -> n-::Kq-扭矩系数/1, n-::Kt-推力系数/1
  n-::Kt-推力系数/1 -> Kt/1
  n-::Kq-扭矩系数/1 -> Kq/1

== system propeller/失败的水流估计模型/螺旋桨模型/螺旋桨工作特性表Backup/If Action Subsystem2 ==
  J' : Inport
  Action Port : ActionPort
  n+::Kq-扭矩系数 : Lookup_n-D  NumberOfTableDimensions=1  BreakpointsForDimension1=[-1,-0.9,-0.8,-0.7,-0.6,-0.5,-0.4,-0.3,-0.2,-0.1,0,0.1,0.2,0.3,0.4,0.5,0.6,0.7,0.8,0.9,1]  BreakpointsForDimension2=[1:3]  Table=[0.019242,0.038636,0.046717,0.049444,0.048333,0.043384,0.043081,0.045202,0.049242,0.051465,0.05197,0.050556,0.046111,0.040556,0.033081,0.024596,0.015543,0.0059848,-0.0059091,-0.013687,-0.016818]  InternalRulePriority=Speed  RndMeth=Simplest  InputSameDT=on
  n+::Kt-推力系数 : Lookup_n-D  NumberOfTableDimensions=1  BreakpointsForDimension1=[-1,-0.9,-0.8,-0.7,-0.6,-0.5,-0.4,-0.3,-0.2,-0.1,0,0.1,0.2,0.3,0.4,0.5,0.6,0.7,0.8,0.9,1]  BreakpointsForDimension2=[1:3]  Table=[0.082134,0.19766,0.30499,0.32898,0.31256,0.2589,0.25511,0.28226,0.35107,0.3738,0.38,0.36686,0.32645,0.26016,0.18188,0.10423,0.04173,-0.018245,-0.05423,-0.065593,-0.06]  InternalRulePriority=Speed  RndMeth=Simplest  InputSameDT=on
  Kt : Outport
  Kq : Outport  Port=2
  wires:
  J'/1 -> n+::Kt-推力系数/1, n+::Kq-扭矩系数/1
  n+::Kt-推力系数/1 -> Kt/1
  n+::Kq-扭矩系数/1 -> Kq/1

== system propeller/失败的水流估计模型/螺旋桨模型/螺旋桨工作特性表Backup/If Action Subsystem3 ==
  J' : Inport
  Action Port : ActionPort
  n-::Kq-扭矩系数 : Lookup_n-D  NumberOfTableDimensions=1  BreakpointsForDimension1=[-1,-0.9,-0.8,-0.7,-0.6,-0.5,-0.4,-0.3,-0.2,-0.1,0,0.1,0.2,0.3,0.4,0.5,0.6,0.7,0.8,0.9,1]  BreakpointsForDimension2=[1:3]  Table=[0.019242,0.016111,0.010354,-0.00035354,-0.014293,-0.025707,-0.034495,-0.041263,-0.046515,-0.051162,-0.05197,-0.051465,-0.049242,-0.045202,-0.043081,-0.043384,-0.04702,-0.049343,-0.045909,-0.038434,-0.016818]  InternalRulePriority=Speed  RndMeth=Simplest  InputSameDT=on
  n-::Kt-推力系数 : Lookup_n-D  NumberOfTableDimensions=1  BreakpointsForDimension1=[-1,-0.9,-0.8,-0.7,-0.6,-0.5,-0.4,-0.3,-0.2,-0.1,0,0.1,0.2,0.3,0.4,0.5,0.6,0.7,0.8,0.9,1]  BreakpointsForDimension2=[1:3]  Table=[0.082134,0.088952,0.080745,0.052336,-0.020896,-0.090341,-0.16989,-0.25764,-0.32014,-0.34981,-0.35676,-0.35549,-0.33409,-0.29015,-0.25379,-0.24924,-0.30379,-0.32197,-0.2947,-0.21894,-0.06]  InternalRulePriority=Speed  RndMeth=Simplest  InputSameDT=on
  Kt : Outport
  Kq : Outport  Port=2
  wires:
  n-::Kq-扭矩系数/1 -> Kq/1
  n-::Kt-推力系数/1 -> Kt/1
  J'/1 -> n-::Kt-推力系数/1, n-::Kq-扭矩系数/1

== system propeller/失败的水流估计模型/预期转速计算/螺旋桨状态模拟/If Action Subsystem ==
  In1 : Inport
  Action Port : ActionPort  ActionPortLabel=else
  Fcn2 : Fcn  Expr=u(1)/(sqrt(u(2)))
  Out1 : Outport
  wires:
  Fcn2/1 -> Out1/1
  In1/1 -> Fcn2/1

== system propeller/失败的水流估计模型/预期转速计算/螺旋桨状态模拟/If Action Subsystem1 ==
  In1 : Inport
  Action Port : ActionPort  ActionPortLabel=if(u1 < 1e-6)
  Fcn2 : Fcn  Expr=abs(u(1))
  Out1 : Outport
  wires:
  In1/1 -> Fcn2/1
  Fcn2/1 -> Out1/1

== system propeller/失败的水流估计模型/预期转速计算/螺旋桨状态模拟/螺旋桨工作特性表 ==
  J' : Inport
  转速 : Inport  Port=2
  If Action Subsystem2 : Subsystem  TreatAsAtomicUnit=on
  If Action Subsystem3 : Subsystem  TreatAsAtomicUnit=on
  If1 : If
  Merge1 : Merge
  Merge2 : Merge
  Kt : Outport
  Kq : Outport  Port=2
  wires:
  If Action Subsystem2/2(Kq) -> Merge2/1
  Merge2/1 -> Kq/1
  If Action Subsystem3/2(Kq) -> Merge2/2
  If Action Subsystem3/1(Kt) -> Merge1/2
  Merge1/1 -> Kt/1
  J'/1 -> If Action Subsystem2/1(J'), If Action Subsystem3/1(J')
  If Action Subsystem2/1(Kt) -> Merge1/1
  转速/1 -> If1/1
  If1/2 -> If Action Subsystem3/Action
  If1/1 -> If Action Subsystem2/Action

== system propeller/失败的水流估计模型/预期转速计算/螺旋桨状态模拟/螺旋桨工作特性表Backup ==
  J' : Inport
  转速 : Inport  Port=2
  If Action Subsystem2 : Subsystem  TreatAsAtomicUnit=on
  If Action Subsystem3 : Subsystem  TreatAsAtomicUnit=on
  If1 : If
  Merge1 : Merge
  Merge2 : Merge
  Kt : Outport
  Kq : Outport  Port=2
  wires:
  If1/1 -> If Action Subsystem2/Action
  If1/2 -> If Action Subsystem3/Action
  转速/1 -> If1/1
  If Action Subsystem2/1(Kt) -> Merge1/1
  J'/1 -> If Action Subsystem3/1(J'), If Action Subsystem2/1(J')
  Merge1/1 -> Kt/1
  If Action Subsystem3/1(Kt) -> Merge1/2
  If Action Subsystem3/2(Kq) -> Merge2/2
  Merge2/1 -> Kq/1
  If Action Subsystem2/2(Kq) -> Merge2/1

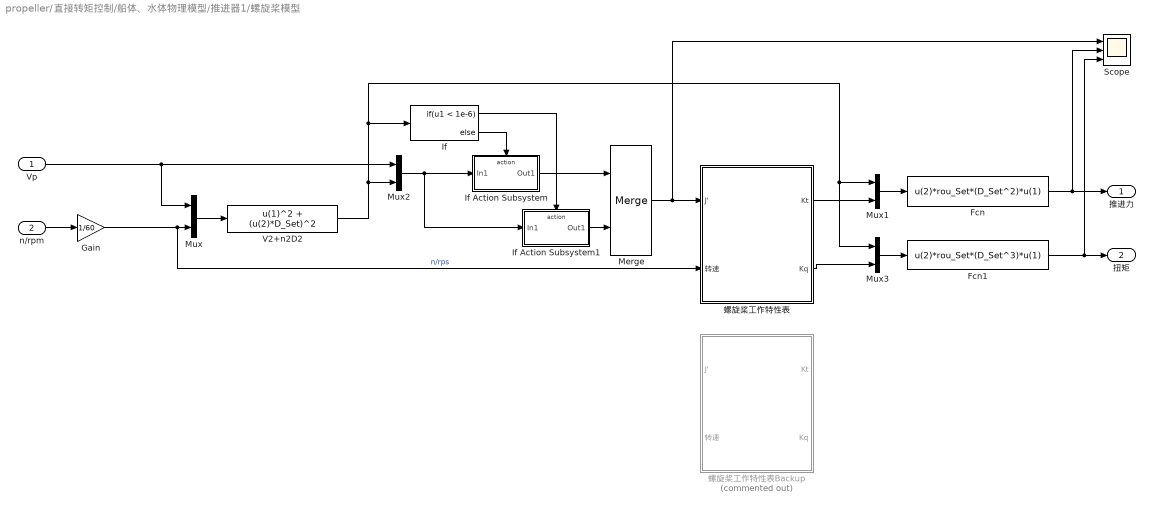
== system propeller/直接转矩控制/船体、水体物理模型/推进器1/螺旋桨模型 ==
  Vp : Inport
  n/rpm : Inport  Port=2
  Fcn : Fcn  Expr=u(2)*rou_Set*(D_Set^2)*u(1)
  Fcn1 : Fcn  Expr=u(2)*rou_Set*(D_Set^3)*u(1)
  Gain : Gain  Gain=1/60
  If : If  IfExpression=u1 < 1e-6
  If Action Subsystem : Subsystem  TreatAsAtomicUnit=on
  If Action Subsystem1 : Subsystem  TreatAsAtomicUnit=on
  Merge : Merge
  Mux{,1..3} (4 alike) : Mux  Inputs=2
  Scope : Scope  NumInputPorts=3
  V2+n2D2 : Fcn  Expr=u(1)^2 + (u(2)*D_Set)^2
  螺旋桨工作特性表 : Subsystem
  螺旋桨工作特性表Backup : Subsystem  Commented=on
  推进力 : Outport
  扭矩 : Outport  Port=2
  wires:
  Fcn/1 -> 推进力/1, Scope/2
  Fcn1/1 -> 扭矩/1, Scope/3
  Mux3/1 -> Fcn1/1
  V2+n2D2/1 -> Mux2/2, Mux1/1, Mux3/1, If/1
  Mux1/1 -> Fcn/1
  螺旋桨工作特性表/2(Kq) -> Mux3/2
  螺旋桨工作特性表/1(Kt) -> Mux1/2
  Merge/1 -> 螺旋桨工作特性表/1(J'), Scope/1
  Mux/1 -> V2+n2D2/1
  If Action Subsystem1/1(Out1) -> Merge/2
  If/1 -> If Action Subsystem1/Action
  Gain/1 -> 螺旋桨工作特性表/2(转速), Mux/2  "n/rps"
  If Action Subsystem/1(Out1) -> Merge/1
  If/2 -> If Action Subsystem/Action
  Vp/1 -> Mux/1, Mux2/1
  n/rpm/1 -> Gain/1
  Mux2/1 -> If Action Subsystem/1(In1), If Action Subsystem1/1(In1)

== system propeller/直接转矩控制/船体、水体物理模型/推进器1/驱动电机 ==
  实际负载扭矩 : Inport
  设定扭矩 : Inport  Port=2
  Gain : Gain  Gain=30/pi
  Integrator : Integrator  LimitOutput=on  UpperSaturationLimit=5000  LowerSaturationLimit=-5000
  Product1 : Product  Inputs=/*
  Saturation : Saturate  UpperLimit=Trq_Max  LowerLimit=-Trq_Max
  Sum1 : Sum  Inputs=|+-
  传感器量化 : Quantizer  QuantizationInterval=Spe_Max/10000
  反馈量滤波 : Subsystem  mask{Frq=25, Order=3}
      mask prompts: Frq "Frq_Set"; Order "Order_Set"
  滞后 : Subsystem  mask{Frq=500, Order=2}
      mask prompts: Frq "Frq_Set"; Order "Order_Set"
  转动惯量 : Constant  Value=J_Set
  通信间隔 : ZeroOrderHold  SampleTime=0.01
  实际转速 : Outport
  转速反馈 : Outport  Port=2
  wires:
  Gain/1 -> 通信间隔/1, 实际转速/1
  反馈量滤波/1(Output) -> 转速反馈/1
  Integrator/1 -> Gain/1  "n_Radps"
  滞后/1(Output) -> Sum1/1
  Product1/1 -> Integrator/1
  Saturation/1 -> 滞后/1(Signal)
  实际负载扭矩/1 -> Sum1/2
  转动惯量/1 -> Product1/1
  传感器量化/1 -> 反馈量滤波/1(Signal)
  Sum1/1 -> Product1/2
  设定扭矩/1 -> Saturation/1
  通信间隔/1 -> 传感器量化/1

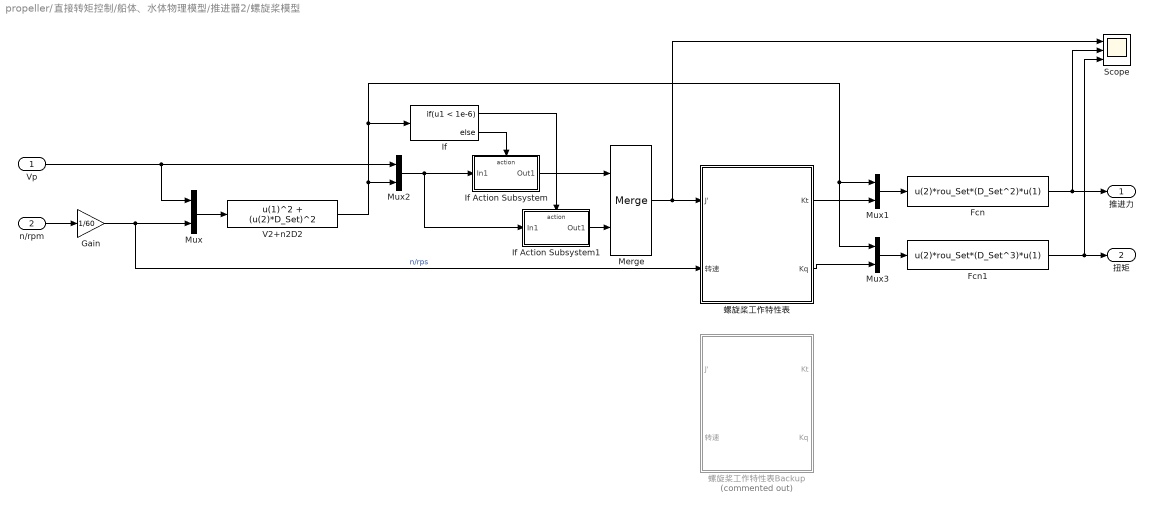
== system propeller/直接转矩控制/船体、水体物理模型/推进器2/螺旋桨模型 ==
  Vp : Inport
  n/rpm : Inport  Port=2
  Fcn : Fcn  Expr=u(2)*rou_Set*(D_Set^2)*u(1)
  Fcn1 : Fcn  Expr=u(2)*rou_Set*(D_Set^3)*u(1)
  Gain : Gain  Gain=1/60
  If : If  IfExpression=u1 < 1e-6
  If Action Subsystem : Subsystem  TreatAsAtomicUnit=on
  If Action Subsystem1 : Subsystem  TreatAsAtomicUnit=on
  Merge : Merge
  Mux{,1..3} (4 alike) : Mux  Inputs=2
  Scope : Scope  NumInputPorts=3
  V2+n2D2 : Fcn  Expr=u(1)^2 + (u(2)*D_Set)^2
  螺旋桨工作特性表 : Subsystem
  螺旋桨工作特性表Backup : Subsystem  Commented=on
  推进力 : Outport
  扭矩 : Outport  Port=2
  wires:
  Mux2/1 -> If Action Subsystem1/1(In1), If Action Subsystem/1(In1)
  n/rpm/1 -> Gain/1
  Vp/1 -> Mux2/1, Mux/1
  If/2 -> If Action Subsystem/Action
  If Action Subsystem/1(Out1) -> Merge/1
  If/1 -> If Action Subsystem1/Action
  If Action Subsystem1/1(Out1) -> Merge/2
  Mux/1 -> V2+n2D2/1
  Merge/1 -> Scope/1, 螺旋桨工作特性表/1(J')
  螺旋桨工作特性表/1(Kt) -> Mux1/2
  螺旋桨工作特性表/2(Kq) -> Mux3/2
  Mux1/1 -> Fcn/1
  V2+n2D2/1 -> If/1, Mux3/1, Mux1/1, Mux2/2
  Mux3/1 -> Fcn1/1
  Fcn1/1 -> Scope/3, 扭矩/1
  Fcn/1 -> Scope/2, 推进力/1
  Gain/1 -> 螺旋桨工作特性表/2(转速), Mux/2  "n/rps"

== system propeller/直接转矩控制/船体、水体物理模型/推进器2/驱动电机 ==
  实际负载扭矩 : Inport
  设定扭矩 : Inport  Port=2
  Gain : Gain  Gain=30/pi
  Integrator : Integrator  LimitOutput=on  UpperSaturationLimit=5000  LowerSaturationLimit=-5000
  Product1 : Product  Inputs=/*
  Saturation : Saturate  UpperLimit=Trq_Max  LowerLimit=-Trq_Max
  Sum1 : Sum  Inputs=|+-
  传感器量化 : Quantizer  QuantizationInterval=Spe_Max/10000
  反馈量滤波 : Subsystem  mask{Frq=25, Order=3}
      mask prompts: Frq "Frq_Set"; Order "Order_Set"
  滞后 : Subsystem  mask{Frq=500, Order=2}
      mask prompts: Frq "Frq_Set"; Order "Order_Set"
  转动惯量 : Constant  Value=J_Set
  通信间隔 : ZeroOrderHold  SampleTime=0.01
  实际转速 : Outport
  转速反馈 : Outport  Port=2
  wires:
  设定扭矩/1 -> Saturation/1
  Sum1/1 -> Product1/2
  转动惯量/1 -> Product1/1
  实际负载扭矩/1 -> Sum1/2
  Saturation/1 -> 滞后/1(Signal)
  Product1/1 -> Integrator/1
  滞后/1(Output) -> Sum1/1
  Integrator/1 -> Gain/1  "n_Radps"
  反馈量滤波/1(Output) -> 转速反馈/1
  Gain/1 -> 实际转速/1, 通信间隔/1
  通信间隔/1 -> 传感器量化/1
  传感器量化/1 -> 反馈量滤波/1(Signal)

== system propeller/直接转矩控制/船速、朝向控制器/前进速度控制/微分 ==
  Err : Inport
  Derivative : Derivative  CoefficientInTFapproximation=0.1
  微分滤波1 : Subsystem  mask{Frq=fc_Set, Order=3}
      mask prompts: Frq "Frq_Set"; Order "Order_Set"
  dErr : Outport
  wires:
  Derivative/1 -> dErr/1
  微分滤波1/1(Output) -> Derivative/1
  Err/1 -> 微分滤波1/1(Signal)

== system propeller/直接转矩控制/船速、朝向控制器/前进速度控制/积分控制 ==
  note: 速度快速增大时积分不增大
      | 速度快速减小时积分不减小
  Error : Inport
  Output : Inport  Port=2
  Derivative : Derivative  CoefficientInTFapproximation=0.1
  Memory : Memory
  Memory1 : Memory
  Product1 : Product  Inputs=3
  Scope : Scope  NumInputPorts=3
  Subsystem : Subsystem
  Zero-Order Hold : ZeroOrderHold  SampleTime=0.01
  Zero-Order Hold1 : ZeroOrderHold  SampleTime=0.01
  Zero-Order Hold2 : ZeroOrderHold  SampleTime=0.01
  输出达到正限幅时积分不再增大 : Subsystem
  输出达到负限幅时积分不再减小 : Subsystem
  开启积分 : Outport
  wires:
  Subsystem/1(启动积分) -> Product1/1, Scope/1  "斜率限制"
  Zero-Order Hold1/1 -> Subsystem/1(dErr)
  Zero-Order Hold2/1 -> Memory1/1
  Derivative/1 -> Zero-Order Hold1/1
  Zero-Order Hold/1 -> Memory/1
  输出达到正限幅时积分不再增大/1(启动积分) -> Product1/2, Scope/2  "正限幅限制"
  输出达到负限幅时积分不再减小/1(启动积分) -> Product1/3, Scope/3  "负限幅限制"
  Output/1 -> Zero-Order Hold2/1
  Product1/1 -> 开启积分/1
  Error/1 -> Zero-Order Hold/1, Derivative/1
  Memory/1 -> 输出达到正限幅时积分不再增大/1(Err), 输出达到负限幅时积分不再减小/1(Err), Subsystem/2(Err)
  Memory1/1 -> 输出达到负限幅时积分不再减小/2(Out), 输出达到正限幅时积分不再增大/2(Out)

== system propeller/直接转矩控制/船速、朝向控制器/右电机控制/角加速度补偿 ==
  转速反馈 : Inport
  Dead Zone : DeadZone  LowerValue=-0.1  UpperValue=0.1  SaturateOnIntegerOverflow=on
  Derivative : Derivative  CoefficientInTFapproximation=1/25
  Gain2 : Gain  Gain=pi/30
  Product1 : Product
  Saturation : Saturate  UpperLimit=Max_Acc  LowerLimit=-Max_Acc
  Transport Delay : TransportDelay  DelayTime=0.01
  滞后1 : Subsystem  mask{Frq=25, Order=10}
      mask prompts: Frq "Frq_Set"; Order "Order_Set"
  滞后2 : Subsystem  mask{Frq=25, Order=10}
      mask prompts: Frq "Frq_Set"; Order "Order_Set"
  转动惯量 : Constant  Value=0.1
  加速消耗的扭矩 : Outport
  wires:
  滞后1/1(Output) -> Saturation/1
  Gain2/1 -> Product1/2
  Saturation/1 -> Gain2/1
  滞后2/1(Output) -> 加速消耗的扭矩/1
  Derivative/1 -> Transport Delay/1
  Product1/1 -> Dead Zone/1
  转动惯量/1 -> Product1/1
  转速反馈/1 -> Derivative/1
  Dead Zone/1 -> 滞后2/1(Signal)
  Transport Delay/1 -> 滞后1/1(Signal)

== system propeller/直接转矩控制/船速、朝向控制器/左电机控制/角加速度补偿 ==
  转速反馈 : Inport
  Dead Zone : DeadZone  LowerValue=-0.1  UpperValue=0.1  SaturateOnIntegerOverflow=on
  Derivative : Derivative  CoefficientInTFapproximation=1/25
  Gain2 : Gain  Gain=pi/30
  Product1 : Product
  Saturation : Saturate  UpperLimit=Max_Acc  LowerLimit=-Max_Acc
  Transport Delay : TransportDelay  DelayTime=0.01
  滞后1 : Subsystem  mask{Frq=25, Order=10}
      mask prompts: Frq "Frq_Set"; Order "Order_Set"
  滞后2 : Subsystem  mask{Frq=25, Order=10}
      mask prompts: Frq "Frq_Set"; Order "Order_Set"
  转动惯量 : Constant  Value=0.1
  加速消耗的扭矩 : Outport
  wires:
  转速反馈/1 -> Derivative/1
  转动惯量/1 -> Product1/1
  Product1/1 -> Dead Zone/1
  Dead Zone/1 -> 滞后2/1(Signal)
  滞后2/1(Output) -> 加速消耗的扭矩/1
  Saturation/1 -> Gain2/1
  Gain2/1 -> Product1/2
  滞后1/1(Output) -> Saturation/1
  Transport Delay/1 -> 滞后1/1(Signal)
  Derivative/1 -> Transport Delay/1

== system propeller/直接转矩控制/船速、朝向控制器/推力解算/扭矩无解 ==
  In1 : Inport
  Action Port : ActionPort  ActionPortLabel=if(u1 < 1e-6)
  Mux : Mux  Inputs=2
  只计算前进推力 : Fcn  Expr=u(1)/(cos(u(5)))*0.5
  Out1 : Outport
  wires:
  In1/1 -> 只计算前进推力/1
  只计算前进推力/1 -> Mux/2, Mux/1
  Mux/1 -> Out1/1
